simulink model "test_h_bridge"  (R2018b)
settings: Solver=VariableStepAuto  StartTime=0.0  StopTime=10.0  RelTol=1e-3
libraries: nesl_utility x4, fl_lib x3, pe_lib x2
settings Model: Creator=Marko  LastModifiedBy=Marko
settings SimscapeCC: SimscapeLogType=all  SimscapeLogLimitData=off

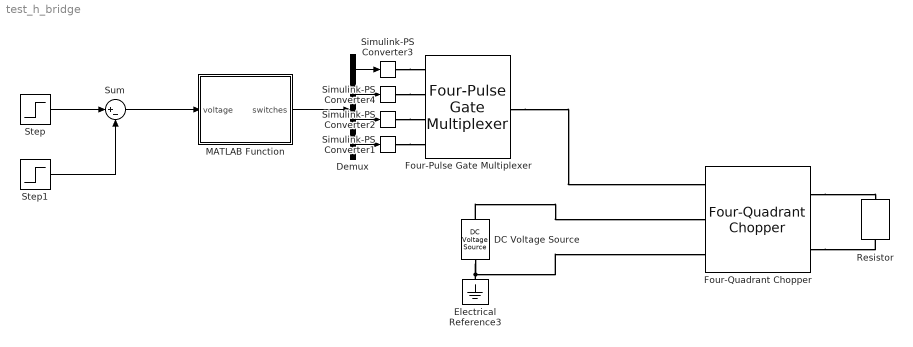
== system test_h_bridge ==
  DC Voltage Source : fl_lib/Electrical/Electrical Sources/DC Voltage Source  v0=250 V
      settings: SourceProductName=Foundation Library
  Demux : Demux
  Electrical Reference3 : fl_lib/Electrical/Electrical Elements/Electrical Reference
      settings: SourceProductName=Foundation Library
  Four-Pulse Gate Multiplexer : pe_lib/Semiconductors/Four-Pulse Gate Multiplexer  R=0 Ohm
      settings: SourceProductName=Simscape Power Systems  SourceProductBaseCode=PS
  Four-Quadrant Chopper : pe_lib/Semiconductors/Four-Quadrant Chopper  device_type=3  Vf=0.8 V  Ron=0.001 Ohm  Rds=0.001 Ohm  Goff=1e-5 1/Ohm  Vth=0.5 V  Vgt=1 V  Vgt_off=-1 V  Ih=1 A  diode_param=2  diode_Vf=0.8 V  diode_Ron=0.001 Ohm  diode_Goff=1e-5 1/Ohm  diode_C=50 nF  diode_iRM=-235 A  diode_iF=300 A  diode_idot=-50 A/us  diode_trr_param=1  diode_trr_factor=3  diode_trr=15 us  diode_Qrr=1500 s*uA  snubber_type=0  Rs=0.1 Ohm  Cs=1e-7 F
      settings: SourceProductName=Simscape Power Systems  SourceProductBaseCode=PS
  MATLAB Function : MATLAB Function  TreatAsAtomicUnit=on  SystemSampleTime=1e-3
  Resistor : fl_lib/Electrical/Electrical Elements/Resistor  R=1000 Ohm  i_specify=off  i_priority=None  i=0 A  i_nominal_specify=off  i_nominal_unit=A  i_nominal_value=1  v_specify=off  v_priority=None  v=0 V  v_nominal_specify=off  v_nominal_unit=V  v_nominal_value=1
  Simulink-PS Converter{1..4} (4 alike) : nesl_utility/Simulink-PS Converter  PhysicalDomain=network_engine_domain  SubClassName=ps_input  LeftPortType=input  RightPortType=output  PseudoPeriodic=off  Frequencies=[]  NoiseDistribution=none  NoiseParameters=[]  Unit=1  AffineConversion=off  FilteringAndDerivatives=filter  SimscapeFilterOrder=2  InputFilterTimeConstant=0.001  UdotUserProvided=0
  Step : Step  Time=31  After=250  SampleTime=0
  Step1 : Step  Time=50  After=250  SampleTime=0
  Sum : Sum  Inputs=|+-
  wires:
  Demux/2 -> Simulink-PS Converter4/1
  Sum/1 -> MATLAB Function/1(voltage)
  Step1/1 -> Sum/2
  Step/1 -> Sum/1
  Demux/3 -> Simulink-PS Converter2/1
  Demux/1 -> Simulink-PS Converter3/1
  MATLAB Function/1(switches) -> Demux/1
  Demux/4 -> Simulink-PS Converter1/1
  connections:
  DC Voltage Source/RConn1 -- Electrical Reference3/LConn1 -- Four-Quadrant Chopper/LConn3
  Simulink-PS Converter1/RConn1 -- Four-Pulse Gate Multiplexer/LConn4
  Simulink-PS Converter3/RConn1 -- Four-Pulse Gate Multiplexer/LConn1
  Simulink-PS Converter2/RConn1 -- Four-Pulse Gate Multiplexer/LConn3
  Simulink-PS Converter4/RConn1 -- Four-Pulse Gate Multiplexer/LConn2
  Four-Quadrant Chopper/RConn1 -- Resistor/LConn1
  Four-Quadrant Chopper/RConn2 -- Resistor/RConn1
  DC Voltage Source/LConn1 -- Four-Quadrant Chopper/LConn2
  Four-Pulse Gate Multiplexer/RConn1 -- Four-Quadrant Chopper/LConn1

== matlab function test_h_bridge/MATLAB Function ==
  data: voltage input; switches output
function switches = pwm(voltage)

s1 = 0;
s2 = 0;
s3 = 0;
s4 = 0;

if(voltage >= 250)
    voltage = 250;
end

if(voltage <= -250)
    voltage = 250;
end

if (voltage == 250)
    s1 = 1;
    s4 = 1;
    s2 = 0;
    s3 = 0;
end

if(voltage == 0)
    s1 = 0;
    s2 = 1;
    s3 = 0;
    s4 = 1;
end


switches = [s1; s2; s3; s4];
